simulink model "psbbuckconv"  (Simulink 6.0)
settings: Solver=ode23tb  SolverMode=SingleTasking  StartTime=0.0  StopTime=0.01  RelTol=1e-3
libraries: powerlib2 x15
settings Model: Creator=patrice  LastModifiedBy=batserve  ExtModeTrigMode=oneshot  ExtModeArmWhenConnect=off  ExtModeAutoUpdateStatusClock=off
settings DataIOCC: LimitDataPoints=off  SignalLoggingName=sigsOut
settings OptimizationCC: BooleanDataType=off
settings DebuggingCC: SolverPrmCheckMsg=none
settings HardwareCC: TargetUnknown=on
settings RTWCC: TemplateMakefile=grt_unix.tmf

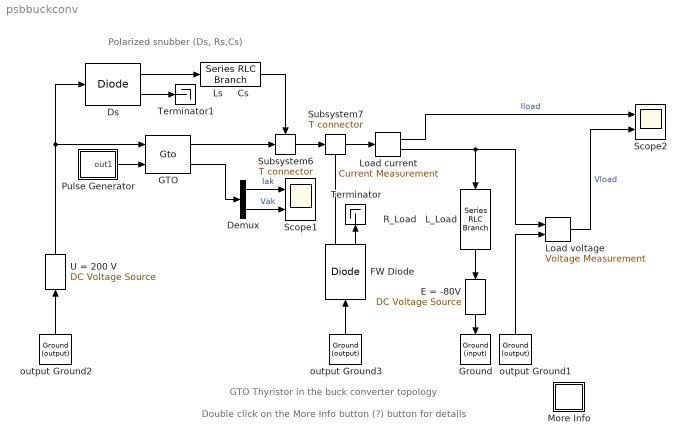
== system psbbuckconv ==
  note: Double click on the More Info button (?) button for details
  note: GTO Thyristor in the buck converter topology
  note: Polarized snubber (Ds, Rs,Cs)
  Demux : Demux  Outputs=2
  Ds : powerlib2/Power Electronics/Diode  Tag=PoWeRsYsTeMbLoCk  Ron=0.01  Lon=1e-6  Vf=0.8  IC=0  Rs=100  Cs=Inf  PSBOutputType=10
  E = -80V : powerlib2/Electrical Sources/DC Voltage Source  Tag=PoWeRsYsTeMbLoCk  Orientation=down  V=-80  mesure=None  PSBOutputType=1
  FW Diode : powerlib2/Power Electronics/Diode  Tag=PoWeRsYsTeMbLoCk  Orientation=up  Ron=0.01  Lon=1e-6  Vf=0.8  IC=0  Rs=100  Cs=0.1e-6  PSBOutputType=10
  GTO : powerlib2/Power Electronics/Gto  Tag=PoWeRsYsTeMbLoCk  Ron=0.01  Lon=1e-6  Vf=1  Tf=10e-6  Tt=20e-6  IC=0  Rs=Inf  Cs=0  PSBOutputType=10
  Ground : powerlib2/Connectors/Ground (input)  Tag=PoWeRsYsTeMbLoCk  Orientation=down
  Load current : powerlib2/Measurements/Current Measurement  Tag=PoWeRsYsTeMmEaSuReMeNt  PhasorSimulation=off  OutputType=Magnitude  PSBOutputType=01  PSBequivalent=0
  Load voltage : powerlib2/Measurements/Voltage Measurement  Tag=PoWeRsYsTeMmEaSuReMeNt  PhasorSimulation=off  OutputType=Magnitude  PSBOutputType=0  PSBequivalent=0
  Ls     Cs : powerlib2/Elements/Series RLC Branch  Tag=PoWeRsYsTeMbLoCk  a=0  b=5e-7  c=2e-6  mesure=None  PSBOutputType=1
  More Info : Subsystem
      mask Display: disp('?')
  Pulse Generator : Subsystem  mask(Pulse Generator){period=1e-3, duty=60, amplitude=1, start=0}
      mask prompts: period "Period (secs):"; duty "Duty cycle (% of period):"; start "Start time:"
      mask help: Pulse Generator
      mask Help: Pulse generator which ensures pulse transitions are hit. Provides a vector of pulses when the height is entered as a vector.  Unmask to see how it works.
      mask Display: plot(0,0,100,100,[95,90,90,75,75,60,60,45,45,30,30,15,15,5],[25,25,75,75,25,25,75,75,25,25,75,75,25,25]);
  R_Load   L_Load : powerlib2/Elements/Series RLC Branch  Tag=PoWeRsYsTeMbLoCk  Orientation=down  a=1  b=5e-03  c=inf  mesure=None  PSBOutputType=1
  Scope1 : Scope  NumInputPorts=2
      settings: TimeRange=0.01  YMin=0~0  YMax=60~300  DataFormat=Array  MaxDataPoints=500000
  Scope2 : Scope  NumInputPorts=2
      settings: TimeRange=0.01  YMin=-50~-100  YMax=50~200  DataFormat=Array  MaxDataPoints=500000
  Subsystem6 : powerlib2/Connectors/T connector  Tag=PoWeRsYsTeMbLoCk  PSBOutputType=1
  Subsystem7 : powerlib2/Connectors/T connector  Tag=PoWeRsYsTeMbLoCk  PSBOutputType=1
  Terminator : Terminator
      settings: Orientation=up
  Terminator1 : Terminator
  U = 200 V : powerlib2/Electrical Sources/DC Voltage Source  Tag=PoWeRsYsTeMbLoCk  Orientation=up  V=200  mesure=None  PSBOutputType=1
  output Ground1 : powerlib2/Connectors/Ground (output)  Tag=PoWeRsYsTeMbLoCk  Orientation=up  PSBOutputType=1
  output Ground2 : powerlib2/Connectors/Ground (output)  Tag=PoWeRsYsTeMbLoCk  Orientation=up  PSBOutputType=1
  output Ground3 : powerlib2/Connectors/Ground (output)  Tag=PoWeRsYsTeMbLoCk  Orientation=up  PSBOutputType=1
  wires:
  Ds/1 -> Ls     Cs/1
  Ls     Cs/1 -> Subsystem6/Enable
  Load current/2 -> Load voltage/1, R_Load   L_Load/1
  output Ground1/1 -> Load voltage/2
  output Ground3/1 -> FW Diode/1
  E = -80V/1 -> Ground/1
  R_Load   L_Load/1 -> E = -80V/1
  U = 200 V/1 -> GTO/1, Ds/1
  Load current/1 -> Scope2/1  "Iload"
  output Ground2/1 -> U = 200 V/1
  Subsystem7/1 -> Load current/1
  Pulse Generator/1(out1) -> GTO/2
  Subsystem6/1 -> Subsystem7/1
  GTO/1 -> Subsystem6/1
  FW Diode/1 -> Subsystem7/Enable
  FW Diode/2 -> Terminator/1
  Ds/2 -> Terminator1/1
  Load voltage/1 -> Scope2/2  "Vload"
  GTO/2 -> Demux/1
  Demux/1 -> Scope1/1  "Iak"
  Demux/2 -> Scope1/2  "Vak"

== system psbbuckconv/More Info ==
  note: A basic polarized snubber circuit ( consisting of Ds, Rs and Cs) is connected across the GTO.
      | The parasitic inductance Ls of the snubber is also taken into consideration.
      | The operating frequency is 1 kHz and the duty cycle is 60%.
  note: This example illustrates use of the GTO-thyristor in the buck converter topology
  note: Circuit Description

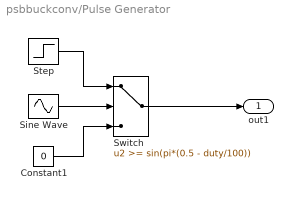
== system psbbuckconv/Pulse Generator ==
  Constant1 : Constant  Value=0
  Sine Wave : Sin  Frequency=2*pi./period  Phase=-2*pi*(start./period + duty/200 - 1/4)  SampleTime=0
  Step : Step  Time=start  After=amplitude  SampleTime=0
  Switch : Switch  Threshold=sin(pi*(0.5 - duty/100))  SaturateOnIntegerOverflow=on  InputSameDT=on
  out1 : Outport  InitialOutput=0
  wires:
  Step/1 -> Switch/1
  Constant1/1 -> Switch/3
  Switch/1 -> out1/1
  Sine Wave/1 -> Switch/2
